simulink model "homework1"  (R2020b)
settings: Solver=FixedStepDiscrete  StartTime=0.0  StopTime=simulation_stop_time  RelTol=1e-3
values from neighbouring files (symbols this model uses):
  sample_time = 1 / input_sample_freq    (= 5e-08)    [data_sample_fp.m]
libraries: hdlsllib x4, simulink x3
settings Model: DataTypeOverride=Off  Creator=yixingli  LastModifiedBy=harsh
settings DataIOCC: LimitDataPoints=on  SaveOutput=off  SignalLogging=off  SaveTime=off
settings OptimizationCC: BlockReduction=off  ConditionallyExecuteInputs=off  DefaultParameterBehavior=Inlined  ExpressionDepthLimit=2147483647  LifeSpan=inf
settings DebuggingCC: AlgebraicLoopMsg=error  UnderspecifiedInitializationDetection=Classic  MergeDetectMultiDrivingBlocksExec=none  SingleTaskRateTransMsg=error  ParameterPrecisionLossMsg=none  AllowSymbolicDim=off  StateNameClashWarn=warning  StrictBusMsg=ErrorOnBusTreatedAsVector  SFUnexpectedBacktrackingDiag=warning  SFNoUnconditionalDefaultTransitionDiag=warning  SFExecutionAtInitializationDiag=none  ArithmeticOperatorsInVariantConditions=warning
settings HardwareCC: ProdBitPerPointer=32  ProdBitPerSizeT=32  ProdBitPerPtrDiffT=32  ProdLargestAtomicFloat=None  ProdIntDivRoundTo=Undefined  ProdEndianess=Unspecified  ProdWordSize=32  ProdHWDeviceType=ASIC/FPGA->ASIC/FPGA  ProdEqTarget=off
settings SFSimCC: SimUseLocalCustomCode=off  CustomCodeUndefinedFunction=UseInterfaceOnly
settings RTWCC: RTWUseLocalCustomCode=off
settings CodeAppCC: StateflowObjectComments=on
settings GRTTargetCC: TargetLangStandard=C89/C90 (ANSI)
settings ConfigComp: CovScope=ReferencedModels  CovMetricSettings=dw  CovSaveCumulativeToWorkspaceVar=on  CovSaveSingleToWorkspaceVar=on  CovExternalEMLEnable=off  CovSFcnEnable=off

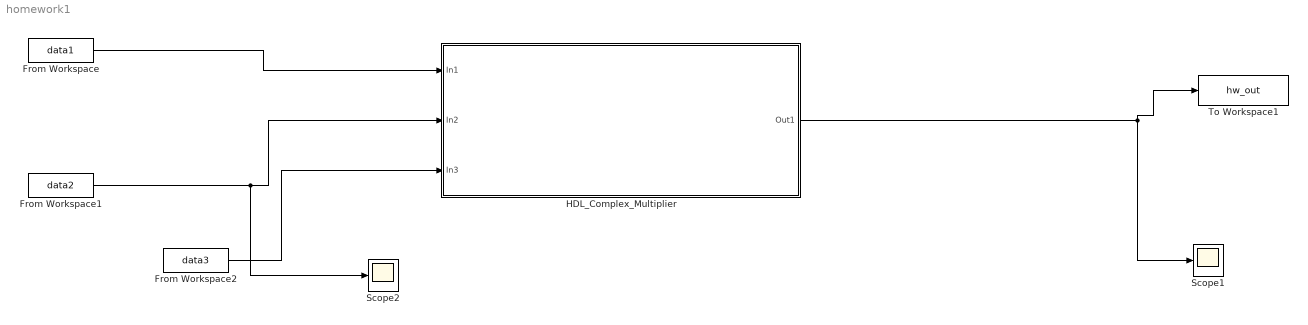
== system homework1 ==
  From Workspace : FromWorkspace  VariableName=data1  SampleTime=sample_time  Interpolate=off  OutputAfterFinalValue=Setting to zero
  From Workspace1 : FromWorkspace  VariableName=data2  SampleTime=sample_time  Interpolate=off  OutputAfterFinalValue=Setting to zero
  From Workspace2 : FromWorkspace  VariableName=data3  SampleTime=sample_time  Interpolate=off  OutputAfterFinalValue=Setting to zero
  HDL_Complex_Multiplier : Subsystem
  Scope1 : Scope
  Scope2 : Scope
  To Workspace1 : ToWorkspace  VariableName=hw_out  SaveFormat=Structure With Time  SampleTime=-1
  wires:
  From Workspace/1 -> HDL_Complex_Multiplier/1(In1)
  From Workspace1/1 -> Scope2/1, HDL_Complex_Multiplier/2(In2)
  HDL_Complex_Multiplier/1(Out1) -> To Workspace1/1, Scope1/1
  From Workspace2/1 -> HDL_Complex_Multiplier/3(In3)

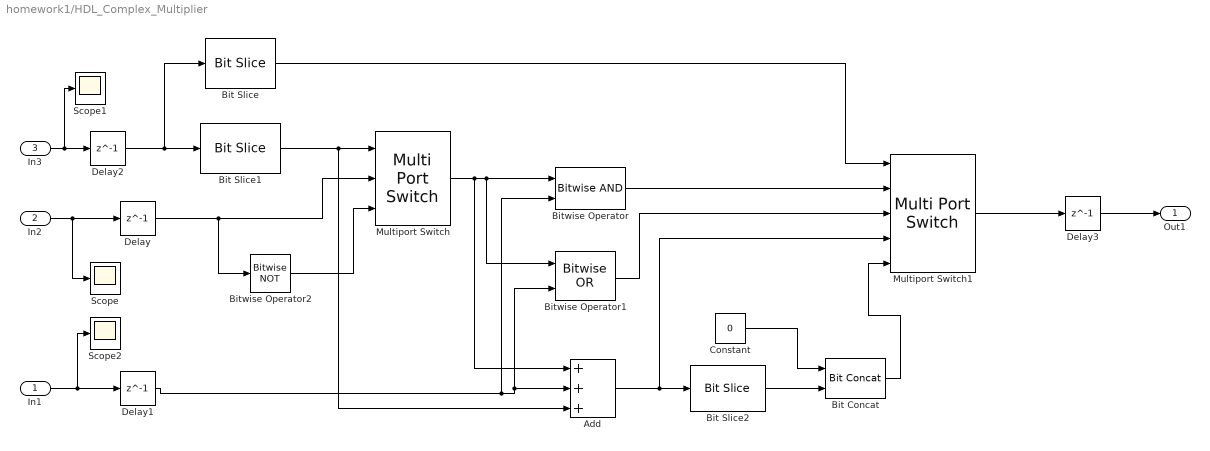
== system homework1/HDL_Complex_Multiplier ==
  In1 : Inport
  In2 : Inport  Port=2
  In3 : Inport  Port=3
  Add : Sum  Inputs=+++  OutDataTypeStr=int64
  Bit Concat : hdlsllib/Logic and Bit Operations/Bit Concat  numInputs=2
  Bit Slice : hdlsllib/Logic and Bit Operations/Bit Slice  lidx=1  ridx=0
      settings: SourceProductBaseCode=SL
  Bit Slice1 : hdlsllib/Logic and Bit Operations/Bit Slice  lidx=2  ridx=2
      settings: SourceProductBaseCode=SL
  Bit Slice2 : hdlsllib/Logic and Bit Operations/Bit Slice  lidx=62  ridx=62
      settings: SourceProductBaseCode=SL
  Bitwise Operator : simulink/Logic and Bit Operations/Bitwise Operator  logicop=AND  UseBitMask=off  NumInputPorts=2  BitMask=bin2dec('11011001')  BitMaskRealWorld=Stored Integer
  Bitwise Operator1 : simulink/Logic and Bit Operations/Bitwise Operator  logicop=OR  UseBitMask=off  NumInputPorts=2  BitMask=bin2dec('11011001')  BitMaskRealWorld=Stored Integer
  Bitwise Operator2 : simulink/Logic and Bit Operations/Bitwise Operator  logicop=NOT  UseBitMask=off  BitMask=bin2dec('11011001')  BitMaskRealWorld=Stored Integer
  Constant : Constant  Value=0  OutMin=0  OutMax=63  OutDataTypeStr=uint64
  Delay{,1..3} (4 alike) : Delay  DelayLength=1  InitialCondition=0
  Multiport Switch : MultiPortSwitch  DataPortOrder=Zero-based contiguous  Inputs=2  zeroidx=on
  Multiport Switch1 : MultiPortSwitch  DataPortOrder=Zero-based contiguous  Inputs=4  zeroidx=on  OutDataTypeStr=int64
  Scope : Scope
  Scope1 : Scope
  Scope2 : Scope
  Out1 : Outport
  wires:
  Delay3/1 -> Out1/1
  Delay/1 -> Bitwise Operator2/1, Multiport Switch/2
  Bitwise Operator2/1 -> Multiport Switch/3
  In3/1 -> Scope1/1, Delay2/1
  Bit Slice/1 -> Multiport Switch1/1
  Multiport Switch1/1 -> Delay3/1
  Delay1/1 -> Bitwise Operator/2, Bitwise Operator1/2, Add/2
  Multiport Switch/1 -> Add/1, Bitwise Operator1/1, Bitwise Operator/1
  Add/1 -> Multiport Switch1/4, Bit Slice2/1
  Constant/1 -> Bit Concat/1
  Bit Slice2/1 -> Bit Concat/2
  Bit Concat/1 -> Multiport Switch1/5
  Bitwise Operator/1 -> Multiport Switch1/2
  Bitwise Operator1/1 -> Multiport Switch1/3
  Delay2/1 -> Bit Slice/1, Bit Slice1/1
  In1/1 -> Scope2/1, Delay1/1
  In2/1 -> Scope/1, Delay/1
  Bit Slice1/1 -> Multiport Switch/1, Add/3
